simulink model "vision_track_point"  (R2018b)
settings: Solver=VariableStepAuto  StartTime=0.0  StopTime=time  RelTol=1e-3
values from neighbouring files (symbols this model uses):
  point = single([x,y])    [Track_point.m]
  position = single(position)    [Track_point.m]
undefined symbols (not defined in the file or in its folder): gray
libraries: visiontextngfix x1, dspvision x1, visionanalysis x1, visionsinks x1
settings Model: Creator=bhawnath.tiwari  LastModifiedBy=yuning.lei
settings SFSimCC: SimUseLocalCustomCode=off
settings RTWCC: RTWUseLocalCustomCode=off
settings CodeAppCC: StateflowObjectComments=on

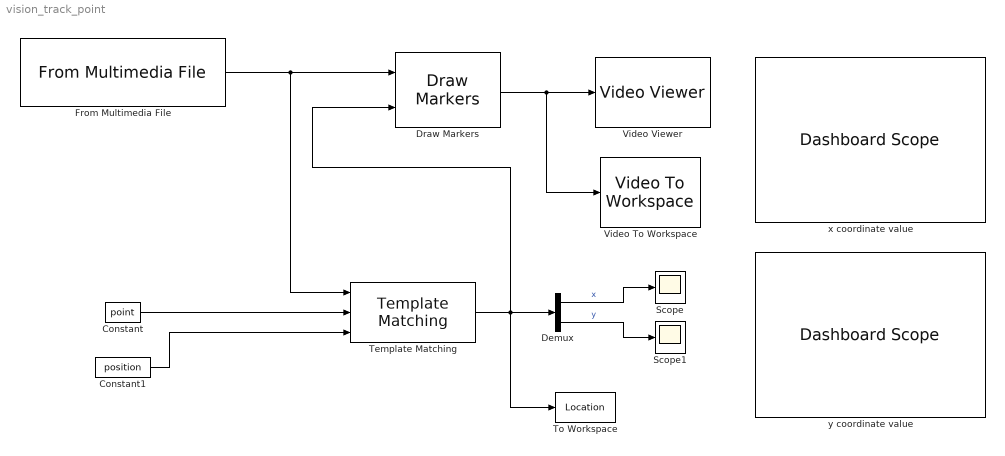
== system vision_track_point ==
  Constant : Constant  Value=point
  Constant1 : Constant  Value=position
  Demux : Demux  Outputs=2
  Draw Markers : visiontextngfix/Draw Markers  shape=Star  size=30  fill=off  fillClrSource=Specify via dialog  display=White  intensity=200  color=[200 255 100]  opacity=0.6  viewport=Entire image  antialiasing=off  inType=Obsolete  imagePorts=One multidimensional signal  prodOutputMode=Binary point scaling  prodOutputWordLength=32  prodOutputFracLength=14  memoryMode=Specify word length  memoryWordLength=16  memoryFracLength=15  roundingMode=Floor  overflowMode=off
      settings: SourceProductName=Computer Vision System Toolbox  SourceProductBaseCode=VP
  From Multimedia File : dspvision/From Multimedia File  inputFilename=g:\Utilisateurs\yuning.lei\Documents\Thèse Yuning\MATLAB\vision_track\pliage01.avi  loop=on  numPlays=inf  outputStreams=Video only  videoDataType=single  audioDataType=int16  inheritSampleTime=on  userDefinedSampleTime=1/30  noAudioOutput=off  isIntensityVideo=off  fourcc=Intensity  colorVideoFormat=One multidimensional signal  outputEOF=off  dataOrg=Column-major  audioFrameSize=1024  computeAudioFrameSize=off  outSamplingMode=Sample based
      settings: SourceProductBaseCode=VP
  Scope : Scope
  Scope1 : Scope
  Template Matching : visionanalysis/Template Matching  metric=Sum of absolute differences  output=Best match location  method=Exhaustive  nMetric=off  nSize=3  roi=on  roiValid=off  roundingMode=Floor  overflowMode=off  prodOutputMode=Binary point scaling  prodOutputWordLength=32  prodOutputFracLength=0  prodOutputSlope=2^0  accumMode=Binary point scaling  accumWordLength=32  accumFracLength=0  accumSlope=2^0  outputSlope=2^0
      settings: SourceProductName=Computer Vision System Toolbox  SourceProductBaseCode=VP
  To Workspace : ToWorkspace  VariableName=Location  SampleTime=-1
      settings: Save2DSignal=2-D array (concatenate along first dimension)
  Video To Workspace : visionsinks/Video To Workspace  VariableName=vout  NumInputs=1  DataLimit=10  DecimationFactor=1  LogFi=off  InPortLabels=R|G|B
      settings: SourceProductName=Computer Vision System Toolbox  SourceProductBaseCode=VP
  Video Viewer : VideoViewer  colormapValue=gray(256)  FigPos=[1921 1038 1920 938]
  x coordinate value : DashboardScope  WebBlockId=21  Ymin=770  Ymax=791
  y coordinate value : DashboardScope  WebBlockId=22  Ymin=330  Ymax=400
  wires:
  From Multimedia File/1 -> Template Matching/1, Draw Markers/1
  Constant/1 -> Template Matching/2
  Constant1/1 -> Template Matching/3
  Template Matching/1 -> To Workspace/1, Demux/1, Draw Markers/2
  Demux/1 -> Scope/1  "x"
  Demux/2 -> Scope1/1  "y"
  Draw Markers/1 -> Video To Workspace/1, Video Viewer/1
